simulink model "saturated_pid"  (R2020a)
settings: Solver=VariableStepAuto  StartTime=0.0  StopTime=20  RelTol=1e-3
settings Model: Creator=USER  LastModifiedBy=USER

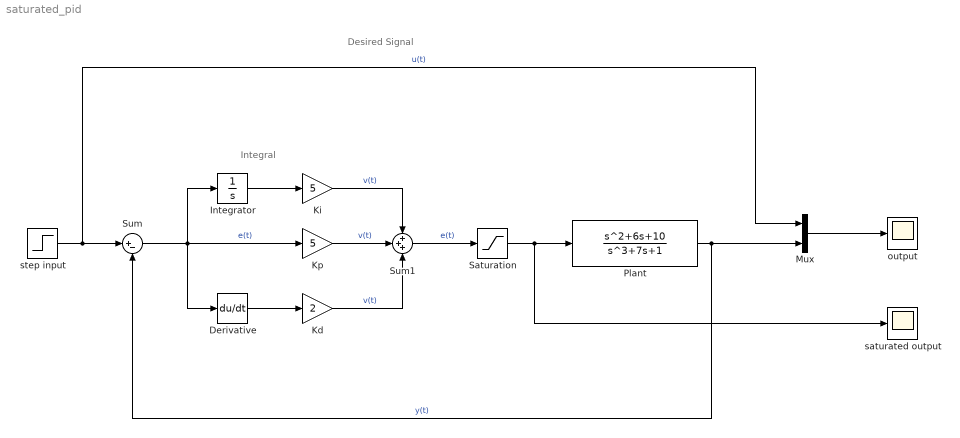
== system saturated_pid ==
  note: Desired Signal
  note: Integral
  Derivative : Derivative
  Integrator : Integrator
  Kd : Gain  Gain=2
  Ki : Gain  Gain=5
  Kp : Gain  Gain=5
  Mux : Mux  Inputs=2
  Plant : TransferFcn  Numerator=[1 6 10]  Denominator=[1 0 7 1]
  Saturation : Saturate  UpperLimit=2  LowerLimit=-2
  Sum : Sum  Inputs=|+-
  Sum1 : Sum  Inputs=+++
  output : Scope
  saturated output : Scope
  step input : Step  After=2  SampleTime=0
  wires:
  step input/1 -> Mux/1, Sum/1  "u(t)"
  Plant/1 -> Mux/2, Sum/2  "y(t)"
  Sum/1 -> Derivative/1, Integrator/1, Kp/1  "e(t)"
  Kp/1 -> Sum1/2  "v(t)"
  Mux/1 -> output/1
  Ki/1 -> Sum1/1  "v(t)"
  Sum1/1 -> Saturation/1  "e(t)"
  Integrator/1 -> Ki/1
  Derivative/1 -> Kd/1
  Kd/1 -> Sum1/3  "v(t)"
  Saturation/1 -> saturated output/1, Plant/1
